simulink model "purepursuit"  (R2023a)
settings: Solver=VariableStepAuto  StartTime=0.0  StopTime=240  RelTol=1e-3
values from neighbouring files (symbols this model uses):
  maxNoise = 0.000001    (= 1e-06)    [main.m]
  minNoise = -0.0000001    (= -1e-07)    [main.m]
libraries: matrix_library x2, robotalgslib x1
settings Model: Creator=ockap  LastModifiedBy=ockap

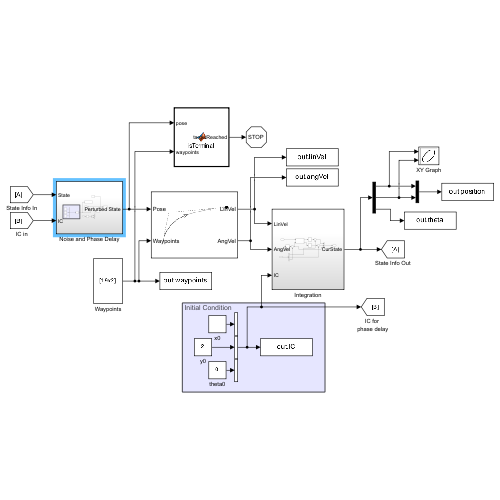
[thumbnail: Simulink's stored preview of the top-level diagram]
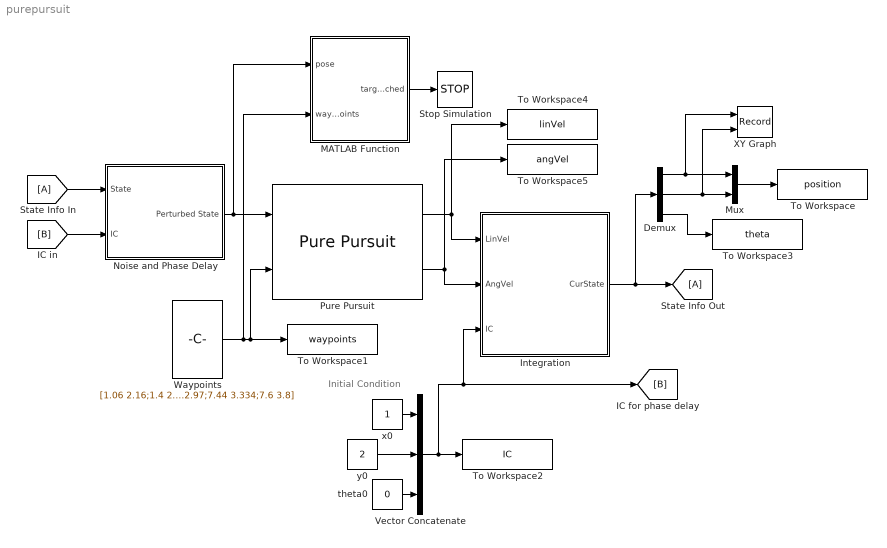
== system purepursuit ==
  note: Initial Condition
  Demux : Demux  Outputs=3
  Integration : Subsystem
  MATLAB Function : MATLAB Function  TreatAsAtomicUnit=on
  Mux : Mux  Inputs=2
  Noise and Phase Delay : Subsystem
  Pure Pursuit : robotalgslib/Pure Pursuit  DesiredLinearVelocity=0.05  MaxAngularVelocity=0.5  LookaheadDistance=0.1  TargetDirPort=off  SimulateUsing=Code generation
      settings: LibrarySourceBlock=robotmobilelib/Pure Pursuit
  State Info In : From
  State Info Out : Goto
  Stop Simulation : Stop
  To Workspace : ToWorkspace  VariableName=position  SaveFormat=Timeseries  SampleTime=-1
  To Workspace1 : ToWorkspace  VariableName=waypoints  SampleTime=-1
      settings: Save2DSignal=2-D array (concatenate along first dimension)
  To Workspace2 : ToWorkspace  VariableName=IC  SampleTime=-1
      settings: Save2DSignal=2-D array (concatenate along first dimension)
  To Workspace3 : ToWorkspace  VariableName=theta  SaveFormat=Timeseries  SampleTime=-1
  To Workspace4 : ToWorkspace  VariableName=linVel  SampleTime=-1
      settings: Save2DSignal=2-D array (concatenate along first dimension)
  To Workspace5 : ToWorkspace  VariableName=angVel  SampleTime=-1
      settings: Save2DSignal=2-D array (concatenate along first dimension)
  Vector Concatenate : Concatenate  NumInputs=3
  Waypoints : Constant  Value=[1.06 2.16;1.4 2.4;1.72 2.744;1.966 3.06;2.336 3.363;2.73 3.45;3.185 3.25;3.74 3.22;4.02 3.64;4.39 4.12;5.02 4.25;5.556 3.96;5.86 3.6;6 3.2;6.37 2.75;6.96 2.58;7.32 2.97;7.44 3.334;7.6 3.8]  VectorParams1D=off  SampleTime=-1
  XY Graph : Record  FileSettingsInternal="{\"entries\":[{\"content\":{\"excelSettings\":{\"content\":{},\"type\":\"Streamout.ExcelSettings\"}},\"type\":\"Streamout.FileSettingStorage\",\"uuid\":\"\"}],\"packageUris\":[\"http:\\/\\/schema.mathworks.com\\/mf0\\/streamout_blocks\\/R2020a\"],\"version\":\"1.0\"}"  Layout=[1 1]  SignalsInternal="{\"entries\":[{\"content\":{\"signals\":[{\"content\":{\"blockPath\":[],\"dimensions\":[1],\"domain\":\"\",\"lineColor\":\"#a2142f\",\"plots\":[1],\"port\":1,\"sid\":[\"\"],\"signalID\":1466,\"signalName\":\"Demux:1\"},\"type\":\"RecordBlkView.Signal\",\"uuid\":\"\"},{\"content\":{\"blockPath\":[],\"dimensions\":[1],\"domain\":\"\",\"lineColor\":\"#139fff\",\"plots\":[1],\"port\":2,\"sid\":[\"\"],\"signalID\":1470,\"signalName\":\"Demux:2\"},\"type\":\"RecordBlkView.Signal\",\"uuid\":\"\"}]},\"type\":\"RecordBlkView.InputSignals\",\"uuid\":\"\"}],\"packageUris\":[\"http:\\/\\/schema.mathworks.com\\/mf0\\/streamout_blocks\\/R2020a\"],\"version\":\"1.0\"}"  VisualizationBindings="{\"xyplotplugin\":{\"info\":[{\"series\":[{\"bindingParametersList\":[{\"parameter\":\"X-Axis\",\"signalID\":1466,\"signalName\":\"Demux:1\"},{\"parameter\":\"Y-Axis\",\"signalID\":1470,\"signalName\":\"Demux:2\"}],\"seriesID\":53499}],\"subplotID\":1}]}}"  CompatibilityTag=XY
  theta0 : Constant  Value=0
  x0 : Constant
  y0 : Constant  Value=2
  wires:
  Demux/1 -> XY Graph/1, Mux/1
  Demux/2 -> XY Graph/2, Mux/2
  Demux/3 -> To Workspace3/1
  Mux/1 -> To Workspace/1
  Vector Concatenate/1 -> To Workspace2/1, [B], Integration/3(IC)
  x0/1 -> Vector Concatenate/1
  Integration/1(CurState) -> State Info Out/1, Demux/1
  y0/1 -> Vector Concatenate/2
  [B] -> Noise and Phase Delay/2(IC)
  theta0/1 -> Vector Concatenate/3
  Pure Pursuit/1 -> To Workspace4/1, Integration/1(LinVel)
  Pure Pursuit/2 -> To Workspace5/1, Integration/2(AngVel)
  Waypoints/1 -> Pure Pursuit/2, To Workspace1/1, MATLAB Function/2(waypoints)
  State Info In/1 -> Noise and Phase Delay/1(State)
  Noise and Phase Delay/1(Perturbed State) -> MATLAB Function/1(pose), Pure Pursuit/1
  MATLAB Function/1(targetReached) -> Stop Simulation/1

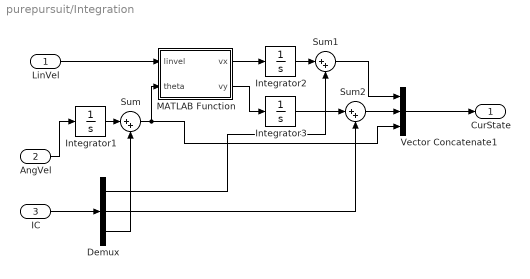
== system purepursuit/Integration ==
  LinVel : Inport
  AngVel : Inport  Port=2
  IC : Inport  Port=3
  Demux : Demux  Outputs=3
  Integrator1 : Integrator
  Integrator2 : Integrator
  Integrator3 : Integrator
  MATLAB Function : MATLAB Function  TreatAsAtomicUnit=on
  Sum : Sum  Inputs=|++
  Sum1 : Sum  Inputs=|++
  Sum2 : Sum  Inputs=|++
  Vector Concatenate1 : Concatenate  NumInputs=3
  CurState : Outport
  wires:
  MATLAB Function/1(vx) -> Integrator2/1
  MATLAB Function/2(vy) -> Integrator3/1
  AngVel/1 -> Integrator1/1
  LinVel/1 -> MATLAB Function/1(linvel)
  Vector Concatenate1/1 -> CurState/1
  Integrator1/1 -> Sum/1
  Demux/3 -> Sum/2
  Integrator2/1 -> Sum1/1
  Demux/1 -> Sum1/2
  Demux/2 -> Sum2/2
  Integrator3/1 -> Sum2/1
  Sum2/1 -> Vector Concatenate1/2
  Sum1/1 -> Vector Concatenate1/1
  IC/1 -> Demux/1
  Sum/1 -> MATLAB Function/2(theta), Vector Concatenate1/3

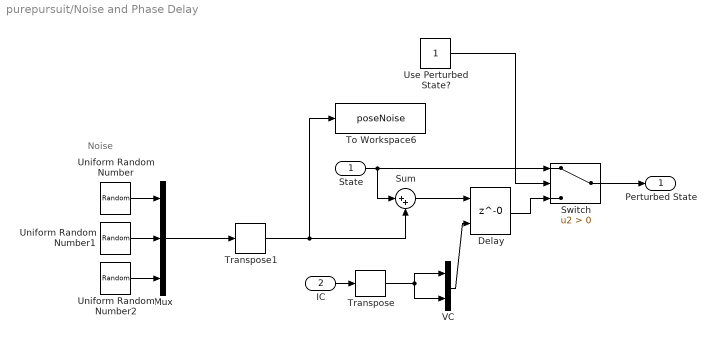
== system purepursuit/Noise and Phase Delay ==
  note: Noise
  State : Inport
  IC : Inport  Port=2
  Delay : Delay  DelayLength=0  InitialConditionSource=Input port  InitialCondition=0  InputProcessing=Columns as channels (frame based)
      settings: InputPortMap=u0,p4
  Mux : Mux  Inputs=3
  Sum : Sum  Inputs=|++
  Switch : Switch  Criteria=u2 > Threshold  SaturateOnIntegerOverflow=off  InputSameDT=off
  To Workspace6 : ToWorkspace  VariableName=poseNoise  SampleTime=-1
      settings: Save2DSignal=2-D array (concatenate along first dimension)
  Transpose : matrix_library/Transpose
  Transpose1 : matrix_library/Transpose
  Uniform Random Number : UniformRandomNumber  Minimum=minNoise  Maximum=maxNoise  SampleTime=0.1
  Uniform Random Number1 : UniformRandomNumber  Minimum=minNoise  Maximum=maxNoise  SampleTime=0.1
  Uniform Random Number2 : UniformRandomNumber  Minimum=minNoise  Maximum=maxNoise  SampleTime=0.1
  Use Perturbed State? : Constant
  VC : Concatenate  Mode=Multidimensional array
  Perturbed State : Outport
  wires:
  IC/1 -> Transpose/1
  Transpose1/1 -> Sum/2, To Workspace6/1
  Transpose/1 -> VC/2, VC/1
  Uniform Random Number2/1 -> Mux/3
  Uniform Random Number1/1 -> Mux/2
  Uniform Random Number/1 -> Mux/1
  Mux/1 -> Transpose1/1
  Sum/1 -> Delay/1
  State/1 -> Switch/1, Sum/1
  Switch/1 -> Perturbed State/1
  Delay/1 -> Switch/3
  Use Perturbed State?/1 -> Switch/2
  VC/1 -> Delay/2

== matlab function purepursuit/Integration/MATLAB Function ==
  data: linvel input; vx output; theta input; vy output
function [vx,vy] = fcn(linvel,theta)
    vx = linvel*cos(theta);
    vy = linvel*sin(theta);
end

== matlab function purepursuit/MATLAB Function ==
  data: pose input; targetReached output; waypoints input
function targetReached = isTerminal(pose,waypoints)
    distance = norm(pose(1:2) - waypoints(end,:));
    targetReached = 0;
    if(distance < 0.03)
        targetReached = 1;
    end
